simulink model "Pointmass_eom_v1_0"  (R2020a)
settings: Solver=ode4  StartTime=0.0  StopTime=simInit.TSIM  FixedStep=simInit.dt  MaxStep=simInit.dt  RelTol=1e-3
InitFcn:
  | close all
values from neighbouring files (symbols this model uses):
  base_windspeed = 12    [initAllSimParams_DE2019.m]
undefined symbols (not defined in the file or in its folder): constr, DE2019, DiscIntNeverNeededParam, ENVMT, Lbooth, loiterStates, params, simInit, T
libraries: simulink x26, simulink_extras x3
(part 3 of 4)

== system Pointmass_eom_v1_0/AirborneSystem/FlightControlSystem/PathFollowingController/FlightOnFlatEarth (Retraction&Loitering)/CalculateAttitudeCmds/FlightPathLoopRetraction_Aerodynamic/FlightpathReferenceModels/SecondOrderReferenceModel_course ==
  y_cmd : Inport
  hedge : Inport  Port=2
  Constant : Constant  Value=omega0_max
  Discrete-Time Integrator : DiscreteIntegrator  SampleTime=-1  LimitOutput=on  UpperSaturationLimit=y_max  LowerSaturationLimit=y_min  ICPrevOutput=DiscIntNeverNeededParam  ICPrevScaledInput=DiscIntNeverNeededParam
  Discrete-Time Integrator1 : DiscreteIntegrator  SampleTime=-1  LimitOutput=on  UpperSaturationLimit=yd_max  LowerSaturationLimit=yd_min  ICPrevOutput=DiscIntNeverNeededParam  ICPrevScaledInput=DiscIntNeverNeededParam
  Gain2 : Gain  Gain=2*zeta0
  Product : Product  Inputs=3
  Product1 : Product
  Saturation : Saturate  UpperLimit=y_max  LowerLimit=y_min
  Saturation1 : Saturate  UpperLimit=y2d_max  LowerLimit=y2d_min
  Sum : Sum  Inputs=|+-
  Sum2 : Sum  Inputs=|+-
  calcualteCourseErrorAndWrap : MATLAB Function  TreatAsAtomicUnit=on
  wrapto2pi : MATLAB Function  TreatAsAtomicUnit=on
  y_ref : Outport  VectorParamsAs1DForOutWhenUnconnected=off
  y_ref_dot : Outport  Port=2  VectorParamsAs1DForOutWhenUnconnected=off
  wires:
  Product1/1 -> Gain2/1
  Constant/1 -> Product1/2, Product/3, Product/1
  Discrete-Time Integrator/1 -> wrapto2pi/1(u)
  Product/1 -> Sum/1
  y_cmd/1 -> Saturation/1
  Discrete-Time Integrator1/1 -> y_ref_dot/1, Product1/1, Sum2/1  "v:_r"
  Sum/1 -> Saturation1/1
  Gain2/1 -> Sum/2
  calcualteCourseErrorAndWrap/1(e_course) -> Product/2
  Saturation1/1 -> Discrete-Time Integrator1/1  "v_dot_r"
  Saturation/1 -> calcualteCourseErrorAndWrap/1(chi_ref)
  Sum2/1 -> Discrete-Time Integrator/1
  hedge/1 -> Sum2/2
  wrapto2pi/1(y) -> calcualteCourseErrorAndWrap/2(chi), y_ref/1

== system Pointmass_eom_v1_0/AirborneSystem/FlightControlSystem/PathFollowingController/FlightOnFlatEarth (Retraction&Loitering)/CalculateAttitudeCmds/FlightPathLoopRetraction_Aerodynamic/FlightpathReferenceModels/SecondOrderReferenceModel_pathangle ==
  y_cmd : Inport
  hedge : Inport  Port=2
  Constant : Constant  Value=omega0_max
  Discrete-Time Integrator : DiscreteIntegrator  SampleTime=-1  LimitOutput=on  UpperSaturationLimit=y_max  LowerSaturationLimit=y_min  ICPrevOutput=DiscIntNeverNeededParam  ICPrevScaledInput=DiscIntNeverNeededParam
  Discrete-Time Integrator1 : DiscreteIntegrator  SampleTime=-1  LimitOutput=on  UpperSaturationLimit=yd_max  LowerSaturationLimit=yd_min  ICPrevOutput=DiscIntNeverNeededParam  ICPrevScaledInput=DiscIntNeverNeededParam
  Gain2 : Gain  Gain=2*zeta0
  Product : Product  Inputs=3
  Product1 : Product
  Saturation : Saturate  UpperLimit=y_max  LowerLimit=y_min
  Saturation1 : Saturate  UpperLimit=y2d_max  LowerLimit=y2d_min
  Sum : Sum  Inputs=|+-
  Sum1 : Sum  Inputs=|+-
  Sum2 : Sum  Inputs=|+-
  y_ref : Outport  VectorParamsAs1DForOutWhenUnconnected=off
  y_ref_dot : Outport  Port=2  VectorParamsAs1DForOutWhenUnconnected=off
  wires:
  Product1/1 -> Gain2/1
  Constant/1 -> Product1/2, Product/3, Product/1
  Product/1 -> Sum/1
  y_cmd/1 -> Saturation/1
  Discrete-Time Integrator1/1 -> y_ref_dot/1, Product1/1, Sum2/1  "v:_r"
  Sum/1 -> Saturation1/1
  Gain2/1 -> Sum/2
  Sum1/1 -> Product/2
  Saturation1/1 -> Discrete-Time Integrator1/1  "v_dot_r"
  Saturation/1 -> Sum1/1
  Sum2/1 -> Discrete-Time Integrator/1
  hedge/1 -> Sum2/2
  Discrete-Time Integrator/1 -> y_ref/1, Sum1/2

== stateflow chart Pointmass_eom_v1_0/AirborneSystem/FlightControlSystem/AirspeedController/Chart1 ==
  state Throttle_Off
    entry: brake_on = 0;
  state Throttle_On
    entry: brake_on = 1;
  (default) -> Throttle_Off
  Throttle_Off -> Throttle_On : [manual_switch_on || brake_flag]
  Throttle_On -> Throttle_Off : [manual_switch_on==0&& brake_flag ==0]
  data: brake_flag input; brake_on output; manual_switch_on input

== stateflow chart Pointmass_eom_v1_0/GroundSystem/StateMachine/StateMachine ==
  state loiter
    entry: flightMode = 1;
    during: F_t_set = calcSetpoint(alpha1,Ft_set_prev,Ft_set_loiter);
    entry: init_throttle_flag = 1;
    entry: sub_flight_state = 1;
  state Traction4 % slowly increase tether force
    entry: flightMode=5;
    during: F_t_set = calcSetpoint(alpha2,Ft_set_prev,Ft_set_loiter);
    exit: init_throttle_flag = 1;
    entry: sub_flight_state = 2;
  state Retraction1
    entry: flightMode=6;
    entry: F_t_set =calcSetpoint(alpha2,F_set_retraction,Ft_set_prev);
    entry: reelin_flag = 1;
    entry: sub_flight_state = 7;
    entry: path_captured_flag = 0;
    %during: F_t_set = calcSetpoint(alpha2,F_set_retraction,Ft_set_prev);
  state Traction2 % slowly increase tether force
    entry: flightMode=5;
    during: F_t_set = calcSetpoint(alpha2,Ft_set_prev,F_T_traction_set);
    exit: init_throttle_flag = 1;
    entry: sub_flight_state = 2;
  state Retraction
    entry: flightMode=6;
    entry: reelin_flag = 1;
    %entry: path_captured_flag = 0;
    during: F_t_set = calcSetpoint(alpha2,F_set_retraction,Ft_set_prev);
    entry: sub_flight_state = 6;
  state Traction1
    entry: flightMode=5;
    during: F_t_set = calcSetpoint(alpha2,Ft_set_prev,F_T_traction_set);
    entry: sub_flight_state = 3;
  state Traction3
    entry: flightMode=5;
    entry: path_captured_flag = 1;
    entry: init_throttle_flag = 0;
    during: F_t_set = calcSetpoint(alpha2,Ft_set_prev,F_T_traction_set);
    entry: sub_flight_state = 4;
  state Trans2Retract
    entry: flightMode=5;
    during: F_t_set = calcSetpoint(alpha2,Ft_set_prev,F_set_retraction);
    entry: sub_flight_state = 5;
  (default) -> loiter
  loiter -> Traction4 % slowly increase tether force : [trigger_kite_mode == 1]
  Traction4 % slowly increase tether force -> Traction2 % slowly increase tether force : [pre_pc_mode_flag==0]
  Retraction1 -> Traction1 : [pos_x_W<x_trigger_transition]
  Retraction -> Retraction1 : [F_t_m<1.1*F_set_retraction]
  Traction2 % slowly increase tether force -> Traction1 : [long_kite>0]
  (junction 286) -> Retraction
  Traction1 -> Traction3 : [cross_track_error < crosstrackerror_condition&&Va>=Vamin]
  Traction3 -> Trans2Retract : [(l_t>l_t_max||init_retraction_flag)]
  Trans2Retract -> (junction 286) [order 1] : [path_parameter_s >= (pi/2+1*pi/180) && path_parameter_s <= pi/2+3*pi/180 && (F_t_m<0.2*F_T_traction_set || l_t>1.2*l_t_max) ]
  (junction 319) -> (junction 286)
  Trans2Retract -> (junction 319) [order 2] : [path_parameter_s >= (3*pi/2+1*pi/180) && path_parameter_s <=3*pi/2+3*pi/180 && (F_t_m<0.2*F_T_traction_set || l_t>1.2*l_t_max)]
  data: Ft_set function_output; alpha1_ function_input; Ft_set_prev_ function_input; F_T_traction_set_ function_input; flightMode output; long_kite input; lat_kite input; l_t input; F_t input; Lbooth parameter; pos_x_W input; pos_y_W input; F_t_set output; F_T_traction_set parameter double; F_set_retraction parameter; a_booth parameter; b_booth parameter; l_t_min parameter; lat_trans parameter; l_t_max parameter; Ft_set_prev input; alpha1 parameter; alpha2 parameter; Va input; lat_init input; traction_trigger input; cross_track_error input; trigger_kite_mode input; init_throttle_flag output size=1; crosstrackerror_condition parameter; Vamin parameter; init_retraction_flag input; Ft_set_loiter parameter; alpha3 parameter; phi0 input; F_t_m input; sub_flight_state output =1; pre_pc_mode_flag input; path_parameter_s input; sim_time input; reelin_flag local; path_captured_flag local; x_trigger_transition input
  function Ft_set = calcSetpoint(alpha1_,Ft_set_prev_, F_T_traction_set_):
    | % Copyright 2020 Delft University of Technology
    | %
    | % Licensed under the Apache License, Version 2.0 (the "License");
    | % you may not use this file except in compliance with the License.
    | % You may obtain a copy of the License at
    | %
    | %      http://www.apache.org/licenses/LICENSE-2.0
    | %
    | % Unless required by applicable law or agreed to in writing, software
    | % distributed under the License is distributed on an "AS IS" BASIS,
    | % WITHOUT WARRANTIES OR CONDITIONS OF ANY KIND, either express or implied.
    | % See the License for the specific language governing permissions and
    | % limitations under the License. 
    | 
    | function Ft_set = calcSetpoint(alpha1_,Ft_set_prev_, F_T_traction_set_)
    |  
    | Ft_set =  alpha1_ * F_T_traction_set_ +(1-alpha1_)*Ft_set_prev_;
    | 
    | end

== stateflow chart Pointmass_eom_v1_0/GroundSystem/StateMachine/checkRetractionCondition ==
  state calcIncrement1
    during: l_tether_predict =l_tether+l_tether-l0;
  state init2
    entry: init_retraction_flag=1;
  state init
    entry: init_retraction_flag=0;
  state calcIncrement
    during: l_tether_predict =l_tether+l_tether-l0;
  state set0length
    entry: l0 = l_tether;
  calcIncrement1 -> (junction 38) : [path_parameter_s >= (3*pi/2-1*pi/180) && path_parameter_s <=3*pi/2+1*pi/180 ]
  init2 -> init : [fm==6]
  (junction 38) -> init2 [order 1] : [l_tether_predict>=l_tether_max*1.15]
  set0length -> calcIncrement1 [order 4] : [path_parameter_s >= (pi/2-1*pi/180) && path_parameter_s <= pi/2+1*pi/180]
  (default) -> init
  set0length -> init [order 2] : [fm==6]
  (junction 38) -> set0length [order 2]
  calcIncrement -> (junction 38) : [path_parameter_s >= (pi/2-1*pi/180) && path_parameter_s <= pi/2+1*pi/180]
  set0length -> init [order 3] : [fm==6]
  init -> set0length : [path_parameter_s >= (pi/2-1*pi/180) && path_parameter_s <= pi/2+1*pi/180 &&fm==5]
  set0length -> calcIncrement [order 1] : [path_parameter_s >= (3*pi/2-1*pi/180) && path_parameter_s <=3*pi/2+1*pi/180 ]
  data: l_tether input; path_parameter_s input; fm input; l0 local; init_retraction_flag output; l_tether_max input; dl local; l_tether_predict local

== matlab function Pointmass_eom_v1_0/AirborneSystem/FlightControlSystem/AirspeedController/Airspeed_Brake/FeedforwardPart ==
  data: gamma input; BF output; nu_V input; ENVMT parameter; Drag_force input; DE2019 parameter
% Copyright 2020 Delft University of Technology
%
% Licensed under the Apache License, Version 2.0 (the "License");
% you may not use this file except in compliance with the License.
% You may obtain a copy of the License at
%
%      http://www.apache.org/licenses/LICENSE-2.0
%
% Unless required by applicable law or agreed to in writing, software
% distributed under the License is distributed on an "AS IS" BASIS,
% WITHOUT WARRANTIES OR CONDITIONS OF ANY KIND, either express or implied.
% See the License for the specific language governing permissions and
% limitations under the License.

function BF = feedforward_brake(gamma, nu_V,  ENVMT, Drag_force, DE2019)
%feedforward_brake - Brake force calculation for velocity decrease
%
% Inputs:
%    gamma      - Path angle (glideslope)
%    nu_V       - Controlled velocity parameter
%    ENVMT      - Environmental characteristics
%    Drag_force	- Drag
%    DE2019     - Aircraft characteristics
%
% Outputs:
%    BF          - Brake force
%
% Example: 
%    BF = feedforward_thrust(gamma, nu_V,  ENVMT, Drag_force, DE2019)
%
% Author: Sebastian Rapp, Ph.D., Revised by: Dylan Eijkelhof, M.Sc.
% Delft University of Technology
% email address: s.rapp@tudelft.nl
% email address: d.eijkelhof@tudelft.nl
% December 2019; Last revision: 06-October-2020

%-------------	BEGIN CODE	--------------

BF = DE2019.mass * ( ENVMT.g * sin(gamma) + nu_V ) + Drag_force; % required thrust

%-------------	 END CODE	--------------
end

== matlab function Pointmass_eom_v1_0/AirborneSystem/FlightControlSystem/AirspeedController/Airspeed_Brake/MATLAB Function ==
  data: F_a_B input; Drag output; AoA input; Lift output
% Copyright 2020 Delft University of Technology
%
% Licensed under the Apache License, Version 2.0 (the "License");
% you may not use this file except in compliance with the License.
% You may obtain a copy of the License at
%
%      http://www.apache.org/licenses/LICENSE-2.0
%
% Unless required by applicable law or agreed to in writing, software
% distributed under the License is distributed on an "AS IS" BASIS,
% WITHOUT WARRANTIES OR CONDITIONS OF ANY KIND, either express or implied.
% See the License for the specific language governing permissions and
% limitations under the License.

function [Drag, Lift] = estimate_draglift(F_a_B, AoA)
%estimate_draglift - Transform drag from B to A reference frame
%
% Inputs:
%    F_a_B     - Aerodynamic forces in body reference frame
%    AoA       - Angle of Attack
%
% Outputs:
%    Drag    - Drag force
%    Lift    - Lift force
%
% Example: 
%    [Drag, Lift] = estimate_draglift(F_a_B, AoA)
%
% Author: Sebastian Rapp, Ph.D., Revised by: Dylan Eijkelhof, M.Sc.
% Delft University of Technology
% email address: s.rapp@tudelft.nl
% email address: d.eijkelhof@tudelft.nl
% December 2019; Last revision: 06-October-2020

%-------------	BEGIN CODE	--------------

F_a_A = [cos(AoA), 0, sin(AoA);
    0, 1, 0; 
    -sin(AoA), 0, cos(AoA)] * F_a_B;

Drag = -F_a_A(1);
Lift = -F_a_A_est(3);

%-------------	 END CODE	--------------

end

== matlab function Pointmass_eom_v1_0/Environment/MATLAB Function ==
  data: vec_W output; vec_O input; wind_direction_rad input
% Copyright 2020 Delft University of Technology
%
% Licensed under the Apache License, Version 2.0 (the "License");
% you may not use this file except in compliance with the License.
% You may obtain a copy of the License at
%
%      http://www.apache.org/licenses/LICENSE-2.0
%
% Unless required by applicable law or agreed to in writing, software
% distributed under the License is distributed on an "AS IS" BASIS,
% WITHOUT WARRANTIES OR CONDITIONS OF ANY KIND, either express or implied.
% See the License for the specific language governing permissions and
% limitations under the License.

function vec_W = transformO2W(vec_O, wind_direction_rad)
%transformO2W - transform inertial reference frame to wind reference frame
%
% Syntax:  vec_W = transformO2W(vec_O, wind_direction_rad)
%
% Inputs:
%    vec_O - Aircraft position in inertial reference frame
%    wind_direction_rad - Wind direction angle compared to intertial
%                         reference frame
%
% Outputs:
%    vec_W  - Propulsive forces in body reference frame
%   
% Example: 
%    vec_W = transformO2W(vec_O, wind_direction_rad)
%
% Other m-files required: none
% Subfunctions: none
% MAT-files required: none
%
% Author: Dylan Eijkelhof, M.Sc.
% Delft University of Technology
% email address: d.eijkelhof@tudelft.nl  
% December 2019; Last revision: 30-September-2019

%------------- BEGIN CODE --------------    

M_WO = [cos(wind_direction_rad), sin(wind_direction_rad), 0;
        sin(wind_direction_rad), -cos(wind_direction_rad), 0;
        0, 0, -1];

vec_W = M_WO*vec_O;
%------------- END CODE --------------   
end

== matlab function Pointmass_eom_v1_0/AirborneSystem/FlightControlSystem/PathFollowingController/FlightOnFlatEarth (Retraction&Loitering)/CalculateAttitudeCmds/FlightPathLoopRetraction_Aerodynamic/FlightPathLoopRetraction/MATLAB Function ==
  data: L_rq output; airdata input; DE2019 parameter; constr parameter
% Copyright 2020 Delft University of Technology
%
% Licensed under the Apache License, Version 2.0 (the "License");
% you may not use this file except in compliance with the License.
% You may obtain a copy of the License at
%
%      http://www.apache.org/licenses/LICENSE-2.0
%
% Unless required by applicable law or agreed to in writing, software
% distributed under the License is distributed on an "AS IS" BASIS,
% WITHOUT WARRANTIES OR CONDITIONS OF ANY KIND, either express or implied.
% See the License for the specific language governing permissions and
% limitations under the License.

function L_rq = fcn(airdata, DE2019,constr)
%fcn - Calculate required lift force
%
% Inputs:
%    airdata     - Airspeed, aoa, sideslip angle
%    DE2019     - Aircraft characteristics
%    constr     - Constraint, maximum lift
%
% Outputs:
%    L_rq    - Required lift
%
% Author: Sebastian Rapp, Ph.D., Revised by: Dylan Eijkelhof, M.Sc.
% Delft University of Technology
% email address: s.rapp@tudelft.nl
% email address: d.eijkelhof@tudelft.nl
% December 2019; Last revision: 06-October-2020

%-------------	BEGIN CODE	--------------

L_rq =  min( 0.5*DE2019.rho_air*DE2019.S_wing*airdata(1)^2 * (DE2019.CL0+DE2019.CL_alpha*airdata(2) ),constr.F_T_max); % max. negative lift

%-------------	 END CODE	--------------
end

== matlab function Pointmass_eom_v1_0/AirborneSystem/FlightControlSystem/AirspeedController/Airspeed_Brake/hedging ==
  data: Drag_force input; gamma input; nu_V output; BF input; ENVMT parameter; DE2019 parameter
% Copyright 2020 Delft University of Technology
%
% Licensed under the Apache License, Version 2.0 (the "License");
% you may not use this file except in compliance with the License.
% You may obtain a copy of the License at
%
%      http://www.apache.org/licenses/LICENSE-2.0
%
% Unless required by applicable law or agreed to in writing, software
% distributed under the License is distributed on an "AS IS" BASIS,
% WITHOUT WARRANTIES OR CONDITIONS OF ANY KIND, either express or implied.
% See the License for the specific language governing permissions and
% limitations under the License.

function nu_V = hedgingV(Drag_force, gamma, BF, ENVMT, DE2019)

%hedgingV
%
% Inputs:
%    Drag_force	- Drag
%    gamma      - Path angle (glideslope)
%    BF         - Brake force
%    ENVMT      - Environmental characteristics
%    DE2019     - Aircraft characteristics
%
% Outputs:
%    nu_V       - Controlled velocity parameter
%
% Example: 
%    nu_V = hedgingV(Drag_force, gamma, BF, ENVMT, DE2019)
%
% Author: Sebastian Rapp, Ph.D., Revised by: Dylan Eijkelhof, M.Sc.
% Delft University of Technology
% email address: s.rapp@tudelft.nl
% email address: d.eijkelhof@tudelft.nl
% December 2019; Last revision: 06-October-2020

%-------------	BEGIN CODE	--------------

nu_V = (BF-Drag_force)/DE2019.mass - ENVMT.g * sin(gamma); 

%-------------	 END CODE	--------------
end

== matlab function Pointmass_eom_v1_0/AirborneSystem/AeroAndPropForces1/Aero_prop ==
  data: F_p_B output; airdata input; DE2019 parameter; delta_t input; F_a_B output; cl_w input; cd_w input; cl_e input; cd_e input; cl_r input; cd_r input
% Copyright 2020 Delft University of Technology
%
% Licensed under the Apache License, Version 2.0 (the "License");
% you may not use this file except in compliance with the License.
% You may obtain a copy of the License at
%
%      http://www.apache.org/licenses/LICENSE-2.0
%
% Unless required by applicable law or agreed to in writing, software
% distributed under the License is distributed on an "AS IS" BASIS,
% WITHOUT WARRANTIES OR CONDITIONS OF ANY KIND, either express or implied.
% See the License for the specific language governing permissions and
% limitations under the License.

function [F_p_B,F_a_B] = simpleAero(airdata, DE2019, delta_t,cl_w,cd_w,cl_e,cd_e,cl_r,cd_r)
%simpleAero - Calculate aerodynamic and propulsive forces
%
% Syntax:  [F_p_B,F_a_B] = simpleAero(airdata, aircraft_struct, delta_t,cl_w,cd_w,cl_e,cd_e,cl_r,cd_r)
%
% Inputs:
%    airdata - Wind speed, angle of attack and side slip angle
%    DE2019 - Aircraft characteristics data structure
%    delta_t - Thrust force
%    cl_w - Lift coefficient wing
%    cd_w - Drag coefficient wing
%    cl_e - Lift coefficient elevator
%    cd_e - Drag coefficient elevator
%    cl_r - Lift coefficient rudder
%    cd_r - Drag coefficient rudder
%
% Outputs:
%    F_p_B  - Propulsive forces in body reference frame
%    F_a_B  - Total aircraft aerodynamic forces in body reference frame
%   
% Example: 
%    [F_p_B,F_a_B] = simpleAero(airdata, DE2019, delta_t,cl_w,cd_w,cl_e,cd_e,cl_r,cd_r)
%
% Other m-files required: none
% Subfunctions: none
% MAT-files required: none
%
% Author: Dylan Eijkelhof, M.Sc.
% Delft University of Technology
% email address: d.eijkelhof@tudelft.nl  
% December 2019; Last revision: 30-September-2019

%------------- BEGIN CODE --------------    
    F_a_B = zeros(3,1);
    F_p_B = zeros(3,1);

    Va = airdata(1);
    alpha = airdata(2);
    beta = airdata(3);    
    Vinf = [Va*cos(alpha)*cos(beta), Va*sin(beta), Va*sin(alpha)*cos(beta)];

    q = 0.5*DE2019.rho_air*Vinf(1)^2;
    
    %% Main Wing
    F_L_main = -cl_w*q*DE2019.S_ref;
    F_D_main = cd_w*q*DE2019.S_ref;
    
    F_x_mw = -F_D_main*cos(alpha) - F_L_main*sin(alpha);
    F_z_mw = F_L_main*cos(alpha);

    %% Elevator
    F_L_el = -cl_e*q*DE2019.S_el;
    F_D_el = -cd_e*q*DE2019.S_el;
    
    F_x_el = F_D_el*cos(alpha)*cos(beta) - F_L_el*sin(alpha)*cos(beta);
    F_z_el = F_L_el*cos(alpha);
   
    %% Rudder
    F_L_vs = 2*cl_r*q*DE2019.S_vs;
    F_D_vs = -2*cd_r*q*DE2019.S_vs;

    F_x_vs = F_D_vs*cos(alpha)*cos(beta);
    F_y_vs = -F_L_vs*cos(beta);
    
    %% Sum of forces
    F_a_B = [F_x_mw+F_x_el+F_x_vs;F_y_vs; F_z_mw+F_z_el];
    
    %% Motor
%     Vd = airdata(1) + delta_t * ( DE2019.k_motor - airdata(1) );
%     Fp_x = 0.5 * 1.225 * DE2019.S_prop * DE2019.C_prop * Vd * (Vd-airdata(1));
    %% No motor, direct feed through
    F_p_B = [delta_t;0;0];
%------------- END CODE -------------- 
end
%

== matlab function Pointmass_eom_v1_0/RequirementModelsAndLogging/MATLAB Function ==
  data: time input; eul input; stop_flag output; eul_old input
function stop_flag = fcn(time, eul,eul_old)
phi = eul(1);
theta = eul(2);
% psi = eul(3);

phi_old = eul_old(1);
theta_old = eul_old(2);
% psi_old = eul_old(3);

if time>40
    if ((phi>pi/2 || phi<-pi/2) && sign(phi) ~= sign(phi_old))
        stop_flag = 1;
    elseif ((theta>pi/2 || theta<-pi/2) && sign(theta) ~= sign(theta_old))
        stop_flag = 1; 
%     elseif ((psi>pi/2 || psi<-pi/2) && sign(psi) ~= sign(psi_old))
%         stop_flag = 1; 
    else
        stop_flag = 0;
    end
else
    stop_flag = 0;
end
end

== stateflow chart Pointmass_eom_v1_0/AirborneSystem/FlightControlSystem/PathFollowingController/FlightOnFlatEarth (Retraction&Loitering)/CalculateAttitudeCmds/FlightPathLoopRetraction_Aerodynamic/FlightPathLoopRetraction/Chart ==
  settings: updateMethod=DISCRETE  sampleTime=0.1
  state ReducedSetforce
    during: fset = 0 ;
    during: t = t + 1;
  state Setforce
    during: fset = Ftset;
    entry: t=0;
  (default) -> Setforce
  Setforce -> ReducedSetforce : [Ftm>Ftset+100]
  ReducedSetforce -> Setforce : [Ftm<Ftset-100]
  data: Ftset input; Ftm input; fset output; t local

== stateflow chart Pointmass_eom_v1_0/AirborneSystem/FlightControlSystem/PathFollowingController/FlightOnFlatEarth (Retraction&Loitering)/GuidanceFlatEarth/LoiteringGuidance/Loiter ==
  state initLoiter
    during: [e_track,course_des,valid_transition_region_flag]  = initLoiterGuidance(kp_course_init, p_x_W,p_y_W, pos_OLoiter_W, R_init_loiter, windDir, Vk, validTransReg_start, validTransReg_end);
  (default) -> (junction 217)
  (junction 217) -> initLoiter : [1]
  data: delta function_output; kp_ function_input; p_x_W_ function_input; p_y_W_ function_input; pos_OLoiter_W_ function_input; R_ function_input; windDirection_rad_ function_input; Vk_ function_input; course_des_ function_output; valid_transition_region_flag_ function_output; validTransReg_start_ function_input; validTransReg_end_ function_input; course_des output; p_y_W input; course_k input; p_x_W input; Vk input; kp_course_init parameter; validTransReg_start parameter; validTransReg_end parameter; pos_OLoiter_W parameter; R_init_loiter parameter; valid_transition_region_flag output; e_track output; reset_flag input; windDir input
  function [delta, course_des_,valid_transition_region_flag_]  = initLoiterGuidance(kp_, p_x_W_,p_y_W_, pos_OLoiter_W_, R_, windDirection_rad_, Vk_, validTransReg_start_, validTransReg_end_):
    | % Copyright 2020 Delft University of Technology
    | %
    | % Licensed under the Apache License, Version 2.0 (the "License");
    | % you may not use this file except in compliance with the License.
    | % You may obtain a copy of the License at
    | %
    | %      http://www.apache.org/licenses/LICENSE-2.0
    | %
    | % Unless required by applicable law or agreed to in writing, software
    | % distributed under the License is distributed on an "AS IS" BASIS,
    | % WITHOUT WARRANTIES OR CONDITIONS OF ANY KIND, either express or implied.
    | % See the License for the specific language governing permissions and
    | % limitations under the License. 
    | 
    | function [delta, course_des_,valid_transition_region_flag_]  = initLoiterGuidance(kp_, p_x_W_,p_y_W_, pos_OLoiter_W_, R_, windDirection_rad_, Vk_, validTransReg_start_, validTransReg_end_) 
    | 
    | %#codegen
    | 
    | %% LOITER GUIDANCE: compare with approach where height and ground track is controlled independently
    | p_W_ = [p_x_W_; p_y_W_; 0];
    | 
    | pos_OLoiter_W_(3) = 0;
    | r_circ_W =  pos_OLoiter_W_;
    | 
    | 
    | p_P =  ( p_W_ - r_circ_W );
    | V = [1, 0; 0, 1; 0, 0];
    | p_P = V*((V'*V)\eye(2))*V'*p_P;
    | p_P = p_P / norm(p_P) * R_;
    | 
    | s_star = atan2( p_P(2), p_P(1) );
    | t_P = [-sin(s_star); cos(s_star); 0]*R_;
    | t_W = t_P;% + r_circ_W;
    | t_O = transformFromWtoO(windDirection_rad_, t_W);
    | 
    | p_proj_W =  p_P + r_circ_W;
    | delta_W = p_W_ - p_proj_W;
    | delta = norm( delta_W );
    | 
    | 
    | epx = t_W/norm(t_W);
    | epy = delta_W/norm(delta_W);
    | epz = cross( epx, epy ); epz = epz/norm(epz);
    | 
    | chi_star = atan2(t_O(2), t_O(1));
    | deltaChi = sign(epz(3))*asin( max( min( delta*kp_/Vk_ ,1),-1) );  %atan2( delta, 0.1*R_ );
    | 
    | course_des_ = chi_star + deltaChi;
    | 
    | bearing_O = [cos(course_des_); sin(course_des_); 0];
    | bearing_W = transformFromOtoW(windDirection_rad_, bearing_O);
    | 
    | if s_star > validTransReg_start_ && s_star < validTransReg_end_
    |     valid_transition_region_flag_ = 1;
    | else
    |     valid_transition_region_flag_ = 0;
    | end

== stateflow chart Pointmass_eom_v1_0/GroundSystem/GroundControl/Chart ==
  note: Counter structure that counts the figures of 8
      | during the traction phase and resets as soon as
      | the retraction phase is triggered
  state counter1
    entry: c=c+1;
    entry: c_out = c;
  state counter2
    entry: c=c+1;
    entry: c_out = c;
  state s1
  state init
    entry:c=-1;
    entry: c_out = c;
  state reset
    entry: c=-1;
    entry: c_out = c;
  state counter3
    entry: c=c+1;
    entry: c_out = c;
  state s4
  state counter
    entry: c=c+1;
    entry: c_out = c;
  reset -> s1 [order 1] : [long>0]
  counter1 -> reset [order 1] : [fm==6]
  counter1 -> counter2 [order 2] : [long<0]
  counter2 -> counter1 [order 1] : [long>0]
  s1 -> counter2 : [long<0]
  init -> s1 [order 1] : [long>0]
  counter2 -> reset [order 2] : [fm==6]
  (default) -> init
  reset -> s4 [order 2] : [long<=0]
  counter3 -> reset [order 1] : [fm==6]
  counter -> reset [order 2] : [fm==6]
  init -> s4 [order 2] : [long<=0]
  s4 -> counter3 : [long>0]
  counter -> counter3 [order 1] : [long>0]
  counter3 -> counter [order 2] : [long<0]
  data: long input; fm input; c_out output; c local

== matlab function Pointmass_eom_v1_0/AirborneSystem/PointMassEOM/PointMassDynamics/PointMassEOM ==
  data: Va input; alpha input; beta input; v_a_dot output; M_OB output; v_k_W output; pos_O output; pos_W output; v_k_B output; chi_k output; gamma_k output; eta_EULER output; v_k_O output; v_w_O input; mu_a input; F_a_B input; F_p_B input; F_t_W input; chi_a input; gamma_a input; long input; lat input; h_tau input; DE2019 parameter; ENVMT parameter; chi_a_dot output; gamma_a_dot output; long_dot output; lat_dot output; h_tau_dot output
% Copyright 2020 Delft University of Technology
%
% Licensed under the Apache License, Version 2.0 (the "License");
% you may not use this file except in compliance with the License.
% You may obtain a copy of the License at
%
%      http://www.apache.org/licenses/LICENSE-2.0
%
% Unless required by applicable law or agreed to in writing, software
% distributed under the License is distributed on an "AS IS" BASIS,
% WITHOUT WARRANTIES OR CONDITIONS OF ANY KIND, either express or implied.
% See the License for the specific language governing permissions and
% limitations under the License.

function [v_a_dot, M_OB, v_k_W, pos_O,pos_W, v_k_B, chi_k, gamma_k,eta_EULER, ...
    v_k_O, chi_a_dot,gamma_a_dot,long_dot,lat_dot,h_tau_dot] = pmEOM(Va, alpha, ...
    beta, v_w_O, mu_a, F_a_B, F_p_B, F_t_W, chi_a, gamma_a, long, lat,h_tau, DE2019, ENVMT)
%pmEOM - Solve adapted equations of motion for a point mass dynamic system
%
% Inputs:
%    Va       - Aircraft velocity component on body x axis
%    alpha    - Aircraft angle of attack
%    beta     - Aircraft side slip angle
%    v_w_O    - Wind velocity at aircraft in inertial reference frame
%    mu_a     - Roll angle aircraft in body reference frame
%    F_a_B    - Aerodynamic forces in body reference frame
%    F_p_B    - Propulsion forces in body reference frame
%    F_t_W    - Tether tension at aircraft in wind reference frame
%    chi_a    - Aerodynamic course heading
%    gamma_a  - Aerodynamic path angle
%    long     - Longtitude, ground station center of earth
%    lat      - Latitude, ground station center of earth
%    h_tau    - Distance from gound station
%    DE2019   - Aircraft parameters in data structure format
%    ENVMT    - Environmental properties
%
% Outputs:
%    v_a_dot        - Aircraft acceleration on body x axis
%    M_OB           - Transformation matrix between inertial and body
%                     reference frames
%    v_k_W          - Kinetic velocity in wind reference frame
%    pos_O          - Aircraft position in inertial reference frame
%    pos_W          - Aircraft position in wind reference frame
%    v_k_B          - Kinetic velocity in body reference frame
%    chi_k          - Kinetic course heading
%    gamma_k        - Kinetic path angle
%    eta_EULER      - Euler angles aircraft
%    v_k_O          - Kinetic velocity in inertial reference frame
%    chi_a_dot      - Time derivative course heading
%    gamma_a_dot    - Time derivative path angle
%    long_dot       - Time derivative longtitude
%    lat_dot        - Time derivative longtitude
%    h_tau_dot      - Time derivative distance from ground station
%
% Example: 
%    [v_a_dot, M_OB, v_k_W, pos_O,pos_W, v_k_B, chi_k, gamma_k,eta_EULER, ...
%     v_k_O, chi_a_dot,gamma_a_dot,long_dot,lat_dot,h_tau_dot] = pmEOM(Va, alpha, ...
%     beta, v_w_O, mu_a, F_a_B, F_p_B, F_t_W, chi_a, gamma_a, long, lat,h_tau, DE2019, ENVMT)
%
% Other m-files required: none
% Subfunctions: none
% MAT-files required: none
%
% Author: Sebastian Rapp, Phd.
% Delft University of Technology
% email address: s.rapp@tudelft.nl  

%------------- BEGIN CODE --------------

%% Pre-allocation of variables for codegen
beta_k= 0;
alpha_k= 0;
chi_k = 0;
gamma_k  = 0;
M_OB = zeros(3); 
eta_EULER = zeros(3,1); 

%% Initiate variables and transformation matrices
M_BA = [cos(alpha), 0, -sin(alpha); 
    0, 1, 0; 
 sin(alpha), -sin(alpha), cos(alpha)];

M_AB = M_BA.';

s_lat = sin(lat); 
s_long = sin(long); 
c_lat = cos(lat); 
c_long = cos(long); 

M_tauW = [-s_lat *c_long, -s_lat *s_long, c_lat;
    -s_long, c_long, 0;
    -c_lat*c_long, -c_lat*s_long, -s_lat ];

xi = ENVMT.windDirection_rad;
M_OW = [cos(xi), sin(xi), 0; 
    sin(xi), -cos(xi), 0; 
    0, 0, -1];
M_WO = M_OW; 

cos_ca = cos(chi_a); 
cos_ga = cos(gamma_a); 
sin_ca = sin(chi_a); 
sin_ga = sin(gamma_a); 

M_AbarO = [cos_ca*cos_ga, sin_ca*cos_ga, -sin_ga; 
    -sin_ca, cos_ca, 0; 
    cos_ca*sin_ga, sin_ca*sin_ga, cos_ga];
M_OAbar = M_AbarO';
M_AbarA = [1,0,0; 
            0, cos(mu_a), -sin(mu_a); 
            0, sin(mu_a), cos(mu_a)];
M_AAbar = M_AbarA';

%%
v_a_O = M_OAbar*[Va;0;0]; 
v_a_B = M_BA*[Va;0;0]; 
v_w_B = M_BA*M_AAbar*M_AbarO*v_w_O;
v_k_B = v_a_B + v_w_B; 
v_k_O = v_a_O + v_w_O; 
v_k_W = M_WO*v_k_O; 
Vk = norm(v_k_B); 

chi_k = atan2( v_k_O(2), v_k_O(1) ); 
gamma_k = -asin( 1/Vk*v_k_O(3) ); 


Ft_Abar = M_AbarO*M_OW*F_t_W;
Fa_Abar = M_AbarA*M_AB*F_a_B; 
Fp_Abar = M_AbarA*M_AB*F_p_B; 
Fg_Abar = M_AbarO*[0;0;DE2019.mass*ENVMT.g];

Ftot_Abar = Ft_Abar + Fg_Abar + Fa_Abar + Fp_Abar; 
x_dot_Abar = 1/DE2019.mass*diag([1,1/(Va*cos_ga),-1/Va]) * Ftot_Abar; 
% states are: Va, chi_a, gamma_a
v_a_dot = x_dot_Abar(1); 
chi_a_dot = x_dot_Abar(2);
gamma_a_dot = x_dot_Abar(3); 

v_k_tau =M_tauW*v_k_W;

long_dot = v_k_tau(2)/( abs(h_tau)*cos(lat));
lat_dot = v_k_tau(1)/abs(h_tau);
h_tau_dot = -v_k_tau(3);

pos_W= [cos(long)*cos(lat); sin(long)*cos(lat); sin(lat)]*h_tau;
pos_O = M_OW*pos_W; 
M_OB = M_OAbar * M_AbarA * M_AB;

%% Calculate euler angles, roll pitch yaw in inertial reference frame
PHI =  atan2( M_OB(3,2), M_OB(3,3) ); 
THETA = -asin( M_OB(3,1) ); 
PSI = atan2( M_OB(2,1), M_OB(1,1) ); 

eta_EULER = [PHI; THETA; PSI];

%------------- END CODE --------------
end

== matlab function Pointmass_eom_v1_0/AirborneSystem/PointMassEOM/MATLAB Function3 ==
  data: v_w_O output; v_w_W input; ENVMT parameter
% Copyright 2020 Delft University of Technology
%
% Licensed under the Apache License, Version 2.0 (the "License");
% you may not use this file except in compliance with the License.
% You may obtain a copy of the License at
%
%      http://www.apache.org/licenses/LICENSE-2.0
%
% Unless required by applicable law or agreed to in writing, software
% distributed under the License is distributed on an "AS IS" BASIS,
% WITHOUT WARRANTIES OR CONDITIONS OF ANY KIND, either express or implied.
% See the License for the specific language governing permissions and
% limitations under the License.

function v_w_O = fcn(v_w_W, ENVMT)



M_OW = [cos(ENVMT.windDirection_rad), sin(ENVMT.windDirection_rad), 0;
        sin(ENVMT.windDirection_rad), -cos(ENVMT.windDirection_rad), 0;
        0, 0, -1];

v_w_O =M_OW*v_w_W;

== matlab function Pointmass_eom_v1_0/AirborneSystem/FlightControlSystem/PathFollowingController/FlightOnFlatEarth (Retraction&Loitering)/CalculateAttitudeCmds/FlightPathLoopRetraction_Aerodynamic/FlightPathLoopRetraction/inversionPathDynamics ==
  data: mu_a_c_old input; f_t input; flightMode input; nu_chi_a input; mu_a_c output; nu_gamma_a input; DE2019 parameter; pos_O input; chi_a input; gamma_a input; airdata input; mu_a input; constr parameter; alpha_a_c output; chi_dot_real output; gamma_dot_real output; ENVMT parameter; L_rq output; Lrq_old input
% Copyright 2020 Delft University of Technology
%
% Licensed under the Apache License, Version 2.0 (the "License");
% you may not use this file except in compliance with the License.
% You may obtain a copy of the License at
%
%      http://www.apache.org/licenses/LICENSE-2.0
%
% Unless required by applicable law or agreed to in writing, software
% distributed under the License is distributed on an "AS IS" BASIS,
% WITHOUT WARRANTIES OR CONDITIONS OF ANY KIND, either express or implied.
% See the License for the specific language governing permissions and
% limitations under the License.

function [mu_a_c,alpha_a_c,chi_dot_real,gamma_dot_real, L_rq] = ...
    InversePathDynamics(mu_a_c_old, f_t, flightMode,nu_chi_a, nu_gamma_a,DE2019, ...
    pos_O, chi_a, gamma_a, airdata, mu_a, constr,ENVMT, Lrq_old)
%InversePathDynamics - Calculated desired roll and pitch angles 
%
% Inputs:
%    mu_a_c_old  - Old desired aerodynamic roll angle
%    f_t         - Corrected tether force set point
%    flightMode  - Flightmode, 6 during retraction
%    nu_chi_a    - Course angle error
%    nu_gamma_a  - Path angle error
%    DE2019      - Aircraft characteristics
%    pos_O       - Aircraft position in inertial reference frame
%    chi_a       - Course angle
%    gamma_a     - Path angle
%    airdata     - Airspeed, aoa and sideslip angle
%    mu_a        - Current roll angle
%    constr      - Dynamic constraints
%    ENVMT       - Environment characteristics
%    L_rq_old    - Old required lift
%
% Outputs:
%    mu_a_c         - Desired roll angle
%    alpha_a_c      - Desired pitch angle
%    chi_dot_real   - Course angle rate of change
%    gamma_dot_real - Path angle rate of change
%    L_rq           - Required lift
%
% Author: Sebastian Rapp, Ph.D., Revised by: Dylan Eijkelhof, M.Sc.
% Delft University of Technology
% email address: s.rapp@tudelft.nl
% email address: d.eijkelhof@tudelft.nl
% December 2019; Last revision: 06-October-2020

%-------------	BEGIN CODE	--------------
%% Initialise parameters for codegen
chi_dot_real = 0;
gamma_dot_real = 0;
push_mode = 0;
mu_a_c = 0;
L_rq = 0;
alpha_a_c = 0;
ddt_v_w_x_O = 0;

%%
c_chi_a = cos(chi_a); 
c_gamma_a = cos(gamma_a); 
s_chi_a = sin(chi_a); 
s_gamma_a = sin(gamma_a); 

Va = airdata(1); 
alpha = airdata(2);

M_AbarO = [ c_chi_a*c_gamma_a, s_chi_a*c_gamma_a, -s_gamma_a; 
    -s_chi_a, c_chi_a, 0; 
    c_chi_a*s_gamma_a, s_chi_a*s_gamma_a, c_gamma_a];

F_g_Abar = M_AbarO * [0;0;DE2019.mass*ENVMT.g];
F_t_Abar = -M_AbarO * pos_O/norm(pos_O)*f_t; 


fy  =  DE2019.mass * ( nu_chi_a * cos(gamma_a) * Va - sin(chi_a)*ddt_v_w_x_O) - F_g_Abar(2) - F_t_Abar(2)  ;
fz =   DE2019.mass  * (nu_gamma_a * Va              - cos(chi_a)*sin(gamma_a)*ddt_v_w_x_O ) + F_g_Abar(3) + F_t_Abar(3);
mu_a_c = atan2(fy,fz);

push_mode = 0;
L_min =  0.5*DE2019.rho_air*DE2019.S_wing*airdata(1)^2 * (DE2019.CL0+DE2019.CL_alpha*constr.alpha_a_min); % max. negative lift

% Recalculation of fy, 
%fy = fz * tan(mu_a); % delay in pull-up
fy = fz * tan(mu_a_c); % leads to pitch then bank behavior.

F_req = min( sqrt( fy^2 + fz^2 ), constr.max_lift );

if abs(mu_a_c)>constr.mu_a_max_retraction && abs(F_req)<abs(L_min) || (fz < 0 && flightMode == 6) % in the retraction phase we want to burn tether force hence it makes sense to fly in push mode.
    mu_a_tmp = mu_a_c + pi; 
    if mu_a_tmp > pi
        du = mod(mu_a_tmp,pi);
        mu_a_tmp = -pi+du;
    elseif mu_a_tmp < -pi
        du = mod(mu_a_tmp,-pi);
        mu_a_tmp = pi+du;
    end
    if abs(mu_a_tmp) <= constr.mu_a_max_retraction || flightMode == 6
        mu_a_c = mu_a_tmp;
        push_mode = 1;
    end
end

mu_a_c = max( min( mu_a_c , constr.mu_a_max_retraction), -constr.mu_a_max_retraction);

%fy = fz * max( min( tan(mu_a_c), 1), -1); % first pull up then bank
fy = fz * tan(mu_a_c);

F_req = min( sqrt( fy^2 + fz^2 ), constr.max_lift );

if push_mode
    L_rq = -F_req;
else
    L_rq = F_req;
end

% hold old bank angle if required lift is very small, avoid agressive
% banking for small absolute values of L i.e. for small values inaccuracies
% like numerical inaccuracies have a large impact on the mu_a_c.
if abs(L_rq) <= 1
    mu_a_c = mu_a_c_old;
end

% for large bank angle changes only adapt the lift if close to the current
% lift. The lontitudional dynamic is faster, hence if we command large bank
% angles this would result in a large lift which would first create a large
% curvature in the longi plane before the actual curvature in the lateral
% plan is achieved.
if abs( mu_a_c - mu_a ) > constr.max_delta_mu
    L_rq = Lrq_old;
end

CL_rq = max( min( 2*L_rq / ( DE2019.rho_air*DE2019.S_wing*airdata(1)^2 ), constr.max_CL), constr.min_CL);
alpha_a_c = max( min( (CL_rq-DE2019.CL0)/DE2019.CL_alpha, constr.alpha_a_max), constr.alpha_a_min); 
CL = max( min( DE2019.CL0+DE2019.CL_alpha*alpha_a_c, constr.max_CL), constr.min_CL);

Lreal = 0.5 * Va^2 * 1.225 * DE2019.S_wing * CL; 
chi_dot_real = 1/cos(gamma_a)/Va/DE2019.mass*(sin(mu_a_c)*Lreal + F_g_Abar(2) + F_t_Abar(2));
gamma_dot_real = -1/Va/DE2019.mass*(-cos(mu_a_c)*Lreal + F_g_Abar(3) + F_t_Abar(3));

%-------------	 END CODE	--------------
end

== matlab function Pointmass_eom_v1_0/AirborneSystem/FlightControlSystem/PathFollowingController/FlightOnFlatEarth (Retraction&Loitering)/CalculateAttitudeCmds/FlightPathLoopRetraction_Aerodynamic/FlightpathReferenceModels/SecondOrderReferenceModel_course/calcualteCourseErrorAndWrap ==
  data: chi_ref input; e_course output; chi input
% Copyright 2020 Delft University of Technology
%
% Licensed under the Apache License, Version 2.0 (the "License");
% you may not use this file except in compliance with the License.
% You may obtain a copy of the License at
%
%      http://www.apache.org/licenses/LICENSE-2.0
%
% Unless required by applicable law or agreed to in writing, software
% distributed under the License is distributed on an "AS IS" BASIS,
% WITHOUT WARRANTIES OR CONDITIONS OF ANY KIND, either express or implied.
% See the License for the specific language governing permissions and
% limitations under the License.

function e_course = course_error(chi_ref, chi)
%course_error - Calculate the error between commanded and actual course angle
%
% Inputs:
%    chi_ref  - Required chi
%    chi      - Actual chi
%
% Outputs:
%    e_course - Course (heading) error
%
% Author: Sebastian Rapp, Ph.D., Revised by: Dylan Eijkelhof, M.Sc.
% Delft University of Technology
% email address: s.rapp@tudelft.nl
% email address: d.eijkelhof@tudelft.nl
% December 2019; Last revision: 06-October-2020

%-------------	BEGIN CODE	--------------
%#codegen
% The vectors are lying in the tangential plane attached to the current
% position on the small earth.
p_bearing_vec =   [cos(chi);         sin(chi);         0];
p_bearing_vec = p_bearing_vec/norm(p_bearing_vec); 
ref_bearing_vec = [cos(chi_ref); sin(chi_ref); 0];
ref_bearing_vec = ref_bearing_vec/norm(ref_bearing_vec); 

e_z = cross( ref_bearing_vec, p_bearing_vec ); 

dot_product = dot( ref_bearing_vec, p_bearing_vec ); 
if dot_product > 1 
    dot_product = 1; 
end
if dot_product < -1 
    dot_product = -1; 
end

e_course = - sign( e_z(3) ) * acos( dot_product );
%-------------	 END CODE	--------------
end

== matlab function Pointmass_eom_v1_0/AirborneSystem/FlightControlSystem/PathFollowingController/FlightOnFlatEarth (Retraction&Loitering)/CalculateAttitudeCmds/FlightPathLoopRetraction_Aerodynamic/FlightpathReferenceModels/SecondOrderReferenceModel_course/wrapto2pi ==
  data: u input; y output
% Copyright 2020 Delft University of Technology
%
% Licensed under the Apache License, Version 2.0 (the "License");
% you may not use this file except in compliance with the License.
% You may obtain a copy of the License at
%
%      http://www.apache.org/licenses/LICENSE-2.0
%
% Unless required by applicable law or agreed to in writing, software
% distributed under the License is distributed on an "AS IS" BASIS,
% WITHOUT WARRANTIES OR CONDITIONS OF ANY KIND, either express or implied.
% See the License for the specific language governing permissions and
% limitations under the License.

function y = wrap_to_2pi(u)
u = mod(u, 2*pi); 
if u > pi 
    du = mod(u,pi);
    y = -pi+du; 
elseif u < -pi 
    du = mod(u,-pi); 
    y = pi+du;
else
    y = u; 
end
end

== matlab function Pointmass_eom_v1_0/AirborneSystem/FlightControlSystem/PathFollowingController/FlightOnFlatEarth (Retraction&Loitering)/CalculateAttitudeCmds/FlightPathLoopRetraction_Aerodynamic/PIController_opt/wrapCourse ==
  data: chi_ref input; e_course output; chi input
% Copyright 2020 Delft University of Technology
%
% Licensed under the Apache License, Version 2.0 (the "License");
% you may not use this file except in compliance with the License.
% You may obtain a copy of the License at
%
%      http://www.apache.org/licenses/LICENSE-2.0
%
% Unless required by applicable law or agreed to in writing, software
% distributed under the License is distributed on an "AS IS" BASIS,
% WITHOUT WARRANTIES OR CONDITIONS OF ANY KIND, either express or implied.
% See the License for the specific language governing permissions and
% limitations under the License.

function e_course = course_error(chi_ref, chi)
%course_error - Calculate the error between commanded and actual course angle
%
% Inputs:
%    chi_ref  - Required chi
%    chi      - Actual chi
%
% Outputs:
%    e_course - Course (heading) error
%
% Author: Sebastian Rapp, Ph.D., Revised by: Dylan Eijkelhof, M.Sc.
% Delft University of Technology
% email address: s.rapp@tudelft.nl
% email address: d.eijkelhof@tudelft.nl
% December 2019; Last revision: 06-October-2020

%-------------	BEGIN CODE	--------------

%#codegen
% The vectors are lying in the tangential plane attached to the current
% position on the small earth.
p_bearing_vec =   [cos(chi);         sin(chi);         0];
p_bearing_vec = p_bearing_vec/norm(p_bearing_vec); 
ref_bearing_vec = [cos(chi_ref); sin(chi_ref); 0];
ref_bearing_vec = ref_bearing_vec/norm(ref_bearing_vec); 

e_z = cross( ref_bearing_vec, p_bearing_vec ); 

dot_product = dot( ref_bearing_vec, p_bearing_vec ); 
if dot_product > 1 
    dot_product = 1; 
end
if dot_product < -1 
    dot_product = -1; 
end

e_course = - sign( e_z(3) ) * acos( dot_product );
%-------------	 END CODE	--------------
end

== stateflow chart Pointmass_eom_v1_0/AirborneSystem/FlightControlSystem/PathFollowingController/FlightOnSphere (Traction)/Select_init_sol_for_pathfollowing ==
  state Pumping
    entry: sol_init = pi/2;
  state Init
    entry: sol_init = x;
  state Pumping1
    entry: sol_init = 3*pi/2;
  (junction 20) -> (junction 21)
  Pumping -> (junction 20) : [fm == 5]
  (junction 21) -> Init
  (default) -> Init
  Init -> (junction 17) : [fm == 6 ]
  (junction 17) -> Pumping [order 1] : [flag_pos_y_W==1]
  (junction 17) -> (junction 12) [order 2] : [flag_pos_y_W==0]
  (junction 24) -> Init
  (junction 12) -> Pumping1
  Pumping1 -> (junction 25) : [fm == 5]
  (junction 25) -> (junction 24)
  data: x input; fm input; sol_init output; flag_pos_y_W input

== matlab function Pointmass_eom_v1_0/AirborneSystem/FlightControlSystem/PathFollowingController/FlightOnFlatEarth (Retraction&Loitering)/CalculateAttitudeCmds/FlightPathLoopRetraction_Aerodynamic/TrafoPathKin2PathAero ==
  data: Va input; beta input; Vg input; v_w_O input; chi_k input; gamma_k input; chi_a output; gamma_a output
% Copyright 2020 Delft University of Technology
%
% Licensed under the Apache License, Version 2.0 (the "License");
% you may not use this file except in compliance with the License.
% You may obtain a copy of the License at
%
%      http://www.apache.org/licenses/LICENSE-2.0
%
% Unless required by applicable law or agreed to in writing, software
% distributed under the License is distributed on an "AS IS" BASIS,
% WITHOUT WARRANTIES OR CONDITIONS OF ANY KIND, either express or implied.
% See the License for the specific language governing permissions and
% limitations under the License.

function [chi_a, gamma_a] = PathKin2PathAero(Va, beta, Vg, v_w_O, chi_k, gamma_k)
%PathKin2PathAero - transform kinetic path angles into aerodynamic path
%                   angles
%
% Inputs:
%    Va         - Aircraft velocity component on body x axis
%    beta       - Aircraft side slip angle
%    Vg         - Kinetic velocity magnitude
%    v_w_O      - Wind velocity at aircraft in inertial reference frame
%    chi_k      - Kinetic course heading
%    gamma_k    - Kinetic path angle
%
% Outputs:
%    chi_a      - Aerodynamic course heading
%    gamma_a 	- Aerodynamic path angle
%
% Example: [chi_a, gamma_a] = fcn(Va, beta, Vg, v_w_O, chi_k, gamma_k)
%
% Other m-files required: none
% Subfunctions: none
% MAT-files required: none
%
% Author: Sebastian Rapp, Phd.
% Delft University of Technology
% email address: s.rapp@tudelft.nl  

%------------- BEGIN CODE --------------
gamma_a = asin( max( min( (Vg*sin(gamma_k)+v_w_O(3))/(Va+1e-9),1), -1) );
chi_a = beta + chi_k - asin( max( min( 1/(Va*cos(gamma_a)) * (v_w_O(1)*(-sin(chi_k))+v_w_O(2)*cos(chi_k)),1), -1) );
%------------- END CODE --------------
end

== stateflow chart Pointmass_eom_v1_0/GroundSystem/GroundControl/Select_init_sol_for_pathfollowing ==
  state Init
    entry: sol_init = x;
  state Pumping
    entry: sol_init = transition_phi;
  (default) -> Init
  Init -> Pumping : [fm == 6]
  data: x input; fm input; sol_init output; transition_phi input

== stateflow chart Pointmass_eom_v1_0/AirborneSystem/FlightControlSystem/PathFollowingController/FlightOnFlatEarth (Retraction&Loitering)/GuidanceFlatEarth/Retraction_Nav/Chart ==
  state no_speed_by_pitch
    during: speed_by_pitch=0;
  state speed_by_pitch
    during: speed_by_pitch=1;
  (default) -> no_speed_by_pitch
  no_speed_by_pitch -> speed_by_pitch : [vkB<v_k_min]
  speed_by_pitch -> no_speed_by_pitch : [vkB>v_k_min+dvk ]
  data: vkB input; speed_by_pitch output; dvk input; v_k_min input
